simulink model "grp_10_simscape_block"  (R2022b)
settings: Solver=FixedStepAuto  StartTime=0.0  StopTime=10  FixedStep=0.005  RelTol=1e-3
undefined symbols (not defined in the file): alphastall, balconyheight, CD0, CD0_fin, CD0_tail, CDmax, CDmax_fin, CDmax_tail, cgoffset, CLmax, CLmax_fin, CLmax_tail, doorheight, doorthickness, doorwidth, finarea, finchord, finlength, finliftcurveslope, finmass, finoffset, finthickness, fuselageheight, fuselagelength, fuselagemass, fuselagewidth, greenwallheight, greyupperwallheight, greywallheight, grounddamping, groundplanedepth, groundplanelength, groundplanewidth, groundstiffness, halllength, hallwidth, initialaltitude, initialpitch, initialroll, initialyaw, kineticfriction, rho, shadowdepth, sidecameraheightoffset, sidecameraoffset, tailarea, tailcameraheightoffset, tailcameraoffset, tailchord, tailliftcurveslope, tailmass, tailoffset, tailsettingangle, tailspan, tailthickness, whitelinedepth, whitelinelength, whitelinewidth, wingarea, wingchord ... (+8)
libraries: sm_lib x164, nesl_utility x127
(part 5 of 5)

== matlab function grp_10_simscape_block/fin aerodynamics/MATLAB Function ==
  data: Vx input; Fx output; Vy input; Vz input; Fz output; My output; CDmax_fin input; CD0_fin input; CLmax_fin input; refarea input; refchord input; rho input; alphastall input; liftcurveslope input
function [Fx,Fz,My] = fcn(Vx, Vy, Vz,CDmax_fin,CD0_fin,CLmax_fin,refarea,refchord,rho,alphastall,liftcurveslope)

%find angle of attack from local wind velocity components
alpha=atan2(Vz, Vx);

%find local wind velocity magnitude
Vref=sqrt(Vx^2 +Vy^2 +Vz^2);

%For post-stall angle of attack, use a simplified trigonemetric model for aerodynamic force and moment coefficients
CL_fin=CLmax_fin*sin(2*alpha);
CD_fin=CD0_fin+CDmax_fin*(sin(alpha))^2;
CM=0; %neglect in baseline model

%This is the pre-stall model; currently just using an approximate
%lift-curve slope of 2*pi (the theoretical maximum), and no attempt to
%model pre-stall drag is included yet:
if alpha*180/pi < alphastall && alpha*180/pi > -alphastall %assumes positive and negative stall anglesd are equal
    CL_fin=liftcurveslope*alpha; 
    %%CD_fin=CD0_fin+(0.06*CL_fin^2);
end

%Find local lift and drag forces in local wind reference frame
lift=0.5*rho*Vref^2*refarea*CL_fin;
drag=0.5*rho*Vref^2*refarea*CD_fin;

%Rotate lift and drag forces from wind reference to local wing reference frame
Fx=drag*cos(alpha)-lift*sin(alpha);
Fy=0;
Fz=drag*sin(alpha)+lift*cos(alpha);

%Find local moment around y axis
My=0.5*rho*Vref^2*refarea*refchord*CM;

end
